simulink subsystem "HVAC_ECU"  (R2021a)
settings: Solver=VariableStepAuto  StartTime=0.0  StopTime=10.0  RelTol=1e-3
libraries: BCM x1
settings Model: Creator=prasad  LastModifiedBy=Sai229

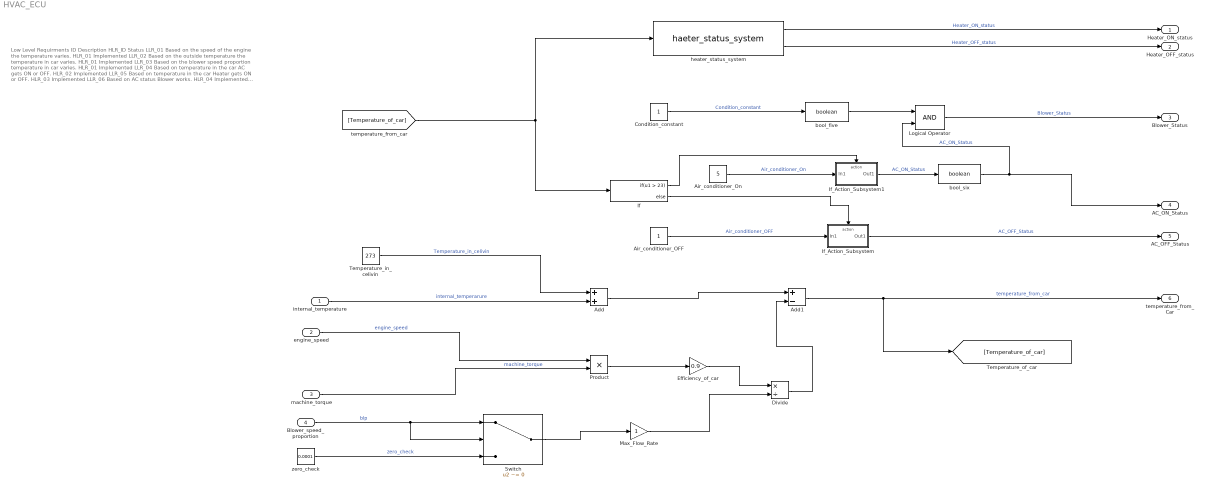
== system HVAC_ECU ==
  note: Low Level Requirments
      | ID
      | Description
      | HLR_ID
      | Status
      |
      | LLR_01
      | Based on the speed of the engine the temperature varies.
      | HLR_01
      | Implemented
      |
      | LLR_02
      | Based on the outside temperature the temperature in car varies.
      | HLR_01
      | Implemented
      |
      | LLR_03
      | Based on the blower speed proportion temperature in car varies.
      | HLR_01
      | Implemented
      |
      | LLR_04
      | Based on temperature in the car AC gets ON or OFF.
      | HLR_02
      | Implemented
      |
      | LLR_05
      | Based on temperature in the car Heater gets ON or OFF.
      | HLR_03
      | Implemented
      |
      | LLR_06
      | Based on AC status Blower works.
      | HLR_04
      | Implemented
      |
      | LOGIC:
      | STEP 1. Taking values of engine temperature and comp Torque and multipled and given to efficiency(gain).
      | STEP 2. Blower speed proportion and given toMaximum flow rate(gain).
      | STEP 3. Both values were given to divide block.
      | STEP 4. Internal Temperature is in degrees and after it converted into kelvin.
      | STEP 5. Subtract of both values, then the temperature will display on the Display block.
      | 1.Based on temperature the AC is getting on.
      | a.If the value(temperature) is greater than 23 then AC should be on.
      | b.Else the AC should be off.
      | 2. Based on AC status Blower Works.
      | 3. Based on temperature the Blower is getting on.
      | a.If the value(temperature) is less than 18 then Heater should be on.
      | b.Else the Heater should be off.
  internal_temperature : Inport
  engine_speed : Inport  Port=2
  machine_torque : Inport  Port=3
  Blower_speed_proportion : Inport  Port=4
  Add : Sum
  Add1 : Sum  Inputs=+-
  Air_conditioner_OFF : Constant
  Air_conditioner_On : Constant  Value=5
  Condition_constant : Constant
  Divide : Product  Inputs=*/
  Efficiency_of_car : Gain  Gain=0.9
  If : If  IfExpression=u1 > 23
  If_Action_Subsystem : Subsystem  TreatAsAtomicUnit=on
  If_Action_Subsystem1 : Subsystem  TreatAsAtomicUnit=on
  Logical Operator : Logic  AllPortsSameDT=off  OutDataTypeStr=boolean
  Max_Flow_Rate : Gain
  Product : Product
  Switch : Switch  Criteria=u2 ~= 0
  Temperature_in_celivin : Constant  Value=273
  bool_five : DataTypeConversion  OutDataTypeStr=boolean
  bool_six : DataTypeConversion  OutDataTypeStr=boolean
  heater_status_system : BCM/haeter_status_system  SystemSampleTime=-1  VariantActivationTime=update diagram  Latency=0  AutoFrameSizeCalculation=off
      settings: SourceProductName=BCM Library
  zero_check : Constant  Value=0.0001
  Heater_ON_status : Outport
  Heater_OFF_status : Outport  Port=2
  Blower_Status : Outport  Port=3
  AC_ON_Status : Outport  Port=4
  AC_OFF_Status : Outport  Port=5
  temperature_from_Car : Outport  Port=6
  wires:
  Add1/1 -> [Temperature_of_car], temperature_from_Car/1  "temperature_from_car"
  If_Action_Subsystem/1(Out1) -> AC_OFF_Status/1  "AC_OFF_Status"
  Divide/1 -> Add1/2
  [Temperature_of_car] -> heater_status_system/1, If/1
  Condition_constant/1 -> bool_five/1  "Condition_constant"
  Efficiency_of_car/1 -> Divide/1
  If/1 -> If_Action_Subsystem1/Action
  Air_conditioner_OFF/1 -> If_Action_Subsystem/1(In1)  "Air_conditioner_OFF"
  Max_Flow_Rate/1 -> Divide/2
  Add/1 -> Add1/1
  Temperature_in_celivin/1 -> Add/1  "Temperature_in_celivin"
  engine_speed/1 -> Product/1  "engine_speed"
  machine_torque/1 -> Product/2  "machine_torque"
  internal_temperature/1 -> Add/2  "internal_temperarure"
  If/2 -> If_Action_Subsystem/Action
  Product/1 -> Efficiency_of_car/1
  Logical Operator/1 -> Blower_Status/1  "Blower_Status"
  Air_conditioner_On/1 -> If_Action_Subsystem1/1(In1)  "Air_conditioner_On"
  heater_status_system/1 -> Heater_ON_status/1  "Heater_ON_status"
  heater_status_system/2 -> Heater_OFF_status/1  "Heater_OFF_status"
  Switch/1 -> Max_Flow_Rate/1
  Blower_speed_proportion/1 -> Switch/2, Switch/1  "blp"
  bool_five/1 -> Logical Operator/1
  If_Action_Subsystem1/1(Out1) -> bool_six/1  "AC_ON_Status"
  bool_six/1 -> AC_ON_Status/1, Logical Operator/2  "AC_ON_Status"
  zero_check/1 -> Switch/3  "zero_check"

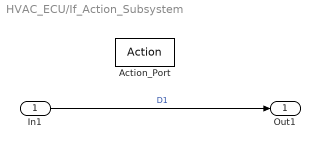
== system HVAC_ECU/If_Action_Subsystem ==
  In1 : Inport
  Action_Port : ActionPort
  Out1 : Outport
  wires:
  In1/1 -> Out1/1  "D1"

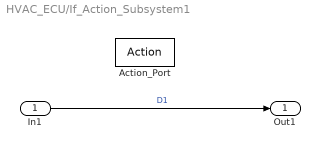
== system HVAC_ECU/If_Action_Subsystem1 ==
  In1 : Inport
  Action_Port : ActionPort
  Out1 : Outport
  wires:
  In1/1 -> Out1/1  "D1"
